simulink model "lorenz_sim"  (R2023b)
settings: Solver=ode45  StartTime=0.0  StopTime=tf  RelTol=1e-6
undefined symbols (not defined in the file): beta, rho, sigma, x0
settings Model: Creator=miqui  LastModifiedBy=miqui

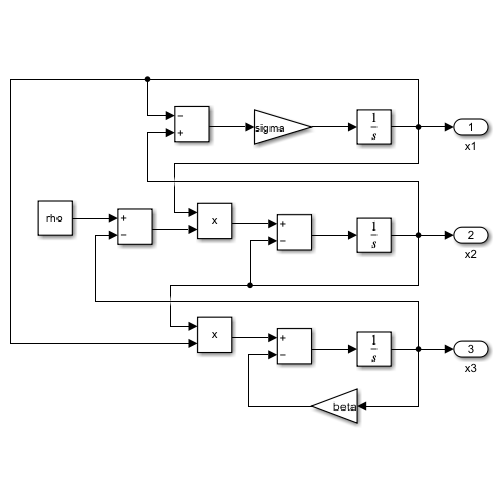
[thumbnail: Simulink's stored preview of the top-level diagram]
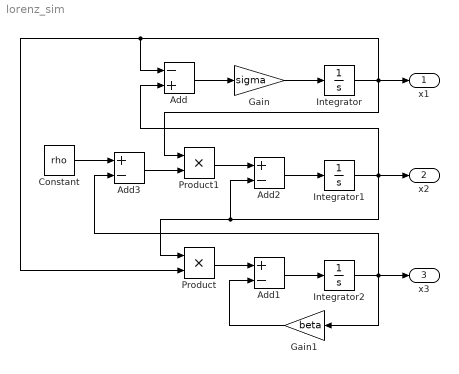
== system lorenz_sim ==
  Add : Sum  Inputs=-+
  Add1 : Sum  Inputs=+-
  Add2 : Sum  Inputs=+-
  Add3 : Sum  Inputs=+-
  Constant : Constant  Value=rho
  Gain : Gain  Gain=sigma
  Gain1 : Gain  Gain=beta
  Integrator : Integrator  InitialCondition=x0(1)
  Integrator1 : Integrator  InitialCondition=x0(2)
  Integrator2 : Integrator  InitialCondition=x0(3)
  Product : Product
  Product1 : Product
  x1 : Outport
  x2 : Outport  Port=2
  x3 : Outport  Port=3
  wires:
  Gain/1 -> Integrator/1
  Add/1 -> Gain/1
  Integrator/1 -> Product/2, Add/1, x1/1, Product1/1
  Integrator1/1 -> Product/1, Add2/2, x2/1, Add/2
  Add1/1 -> Integrator2/1
  Integrator2/1 -> Gain1/1, Add3/2, x3/1
  Gain1/1 -> Add1/2
  Product/1 -> Add1/1
  Add2/1 -> Integrator1/1
  Product1/1 -> Add2/1
  Add3/1 -> Product1/2
  Constant/1 -> Add3/1
